simulink model "torqueWalkingMPC"  (Simulink 8.9)
settings: Solver=FixedStepDiscrete  StartTime=0.0  StopTime=Config.t_end  FixedStep=Config.t_step  RelTol=1e-3  EnableMultiTasking=on
InitFcn:
  | cd(fileparts(which(bdroot)));
  | initTorqueWalking;
undefined symbols (not defined in the file or in its folder): biasVectorConstraint_feet, Config, ConstraintMatrix_feet, DiscIntNeverNeededParam, Gains, ROBOT_DOF, Sat
libraries: WBToolboxLibrary x93
(part 3 of 3)

== system torqueWalkingMPC/Dynamics and Kinematics/Inverse Kinematics/QP-Based Inverse Kinematics/inverse kinematics integration ==
  nuDot : Inport
  nu_0 : Inport  Port=2
  q_0 : Inport  Port=3
  Compute Base Pose Derivative : MATLAB Function  TreatAsAtomicUnit=on
  Demux : Demux  Outputs=[7;ROBOT_DOF]
  Demux1 : Demux  Outputs=[6; ROBOT_DOF]
  Demux2 : Demux  Outputs=[16; ROBOT_DOF]
  Integrate nu : DiscreteIntegrator  InitialConditionSource=external  SampleTime=Config.t_step  ICPrevOutput=DiscIntNeverNeededParam  ICPrevScaledInput=DiscIntNeverNeededParam
  Integrate nuDot : DiscreteIntegrator  InitialConditionSource=external  SampleTime=Config.t_step  ICPrevOutput=DiscIntNeverNeededParam  ICPrevScaledInput=DiscIntNeverNeededParam
  Matrix Concatenate : Concatenate  NumInputs=3  Mode=Multidimensional array  ConcatenateDimension=2
  Mux : Mux  Inputs=2
  Mux1 : Mux  Inputs=2
  Mux2 : Mux  Inputs=2
  Reshape : Reshape
  Reshape1 : Reshape  OutputDimensionality=Customize  OutputDimensions=[4;4]
  Rewrite Base Pose as pos+quat : MATLAB Function  TreatAsAtomicUnit=on
  Rewrite Base Pose as transformation matrix : MATLAB Function  TreatAsAtomicUnit=on
  Selector3 : Selector  InputPortWidth=ROBOT_DOF+6  IndexOptions=Index vector (dialog)  Indices=[7:ROBOT_DOF+6]  OutputSizes=1
  Selector4 : Selector  InputPortWidth=ROBOT_DOF+6  IndexOptions=Index vector (dialog)  Indices=[7:ROBOT_DOF+6]  OutputSizes=1
  nu : Outport
  q : Outport  Port=2
  s_sDot_sDDot_des : Outport  Port=3
  wires:
  nu_0/1 -> Integrate nuDot/2
  nuDot/1 -> Selector4/1, Integrate nuDot/1
  Demux/1 -> Rewrite Base Pose as transformation matrix/1(pose_b), Compute Base Pose Derivative/1(pose_b)
  Integrate nu/1 -> Demux/1
  Compute Base Pose Derivative/1(pose_bDot) -> Mux/1
  Demux1/2 -> Mux/2
  Matrix Concatenate/1 -> s_sDot_sDDot_des/1
  Selector3/1 -> Matrix Concatenate/2
  Selector4/1 -> Matrix Concatenate/3
  Demux/2 -> Matrix Concatenate/1, Mux1/2
  Mux/1 -> Integrate nu/1
  Integrate nuDot/1 -> Selector3/1, nu/1, Demux1/1
  Rewrite Base Pose as transformation matrix/1(w_H_b) -> Reshape/1
  Reshape/1 -> Mux1/1
  Mux1/1 -> q/1
  Demux1/1 -> Compute Base Pose Derivative/2(nu_b)
  q_0/1 -> Demux2/1
  Demux2/1 -> Reshape1/1
  Reshape1/1 -> Rewrite Base Pose as pos+quat/1(w_H_b_0)
  Rewrite Base Pose as pos+quat/1(pose_b_0) -> Mux2/1
  Demux2/2 -> Mux2/2
  Mux2/1 -> Integrate nu/2

== system torqueWalkingMPC/Dynamics and Kinematics/Task Accelerations/ComputeTasksPoseAndVelocity/Task position and orientation ==
  s : Inport
  w_H_b : Inport  Port=2
  CoM : WBToolboxLibrary/wholeBodyModel/Kinematics/Forward Kinematics  frameName=Frames.COM  robotName=WBT_robotName  localName=WBT_modelName  wbiFile=WBT_wbiFilename  wbiList=WBT_wbiList
  LFoot : WBToolboxLibrary/wholeBodyModel/Kinematics/Forward Kinematics  frameName=Frames.LEFT_FOOT  robotName=WBT_robotName  localName=WBT_modelName  wbiFile=WBT_wbiFilename  wbiList=WBT_wbiList
  RFoot : WBToolboxLibrary/wholeBodyModel/Kinematics/Forward Kinematics  frameName=Frames.RIGHT_FOOT  robotName=WBT_robotName  localName=WBT_modelName  wbiFile=WBT_wbiFilename  wbiList=WBT_wbiList
  rotational task : WBToolboxLibrary/wholeBodyModel/Kinematics/Forward Kinematics  frameName=Frames.ROT_TASK_LINK  robotName=WBT_robotName  localName=WBT_modelName  wbiFile=WBT_wbiFilename  wbiList=WBT_wbiList
  w_H_CoM : Outport
  w_H_l_sole : Outport  Port=2
  w_H_r_sole : Outport  Port=3
  w_H_rot_task : Outport  Port=4
  wires:
  s/1 -> rotational task/2, RFoot/2, LFoot/2, CoM/2
  w_H_b/1 -> rotational task/1, CoM/1, LFoot/1, RFoot/1
  CoM/1 -> w_H_CoM/1
  LFoot/1 -> w_H_l_sole/1
  RFoot/1 -> w_H_r_sole/1
  rotational task/1 -> w_H_rot_task/1

== system torqueWalkingMPC/Robot State and References/Smooth References /Smooth Reference Orientations/Compose Smoothed References ==
  omegaDot_LFoot : Inport
  omegaDot_RFoot : Inport  Port=2
  omegaDot_rot_task : Inport  Port=3
  w_R_rot_task : Inport  Port=4
  w_R_RFoot : Inport  Port=5
  w_R_LFoot : Inport  Port=6
  omega_LFoot : Inport  Port=7
  omega_RFoot : Inport  Port=8
  omega_rot_task : Inport  Port=9
  Matrix Concatenate1 : Concatenate  NumInputs=3  Mode=Multidimensional array  ConcatenateDimension=2
  Matrix Concatenate2 : Concatenate  NumInputs=3  Mode=Multidimensional array  ConcatenateDimension=2
  Matrix Concatenate6 : Concatenate  NumInputs=3  Mode=Multidimensional array  ConcatenateDimension=2
  orient_vel_acc_LFoot_des : Outport
  orient_vel_acc_RFoot_des : Outport  Port=2
  orient_vel_acc_rot_task_des : Outport  Port=3
  wires:
  w_R_LFoot/1 -> Matrix Concatenate6/1
  Matrix Concatenate6/1 -> orient_vel_acc_LFoot_des/1
  Matrix Concatenate2/1 -> orient_vel_acc_rot_task_des/1
  Matrix Concatenate1/1 -> orient_vel_acc_RFoot_des/1
  omega_LFoot/1 -> Matrix Concatenate6/2
  omegaDot_LFoot/1 -> Matrix Concatenate6/3
  omegaDot_RFoot/1 -> Matrix Concatenate1/3
  omega_RFoot/1 -> Matrix Concatenate1/2
  w_R_RFoot/1 -> Matrix Concatenate1/1
  omegaDot_rot_task/1 -> Matrix Concatenate2/3
  omega_rot_task/1 -> Matrix Concatenate2/2
  w_R_rot_task/1 -> Matrix Concatenate2/1

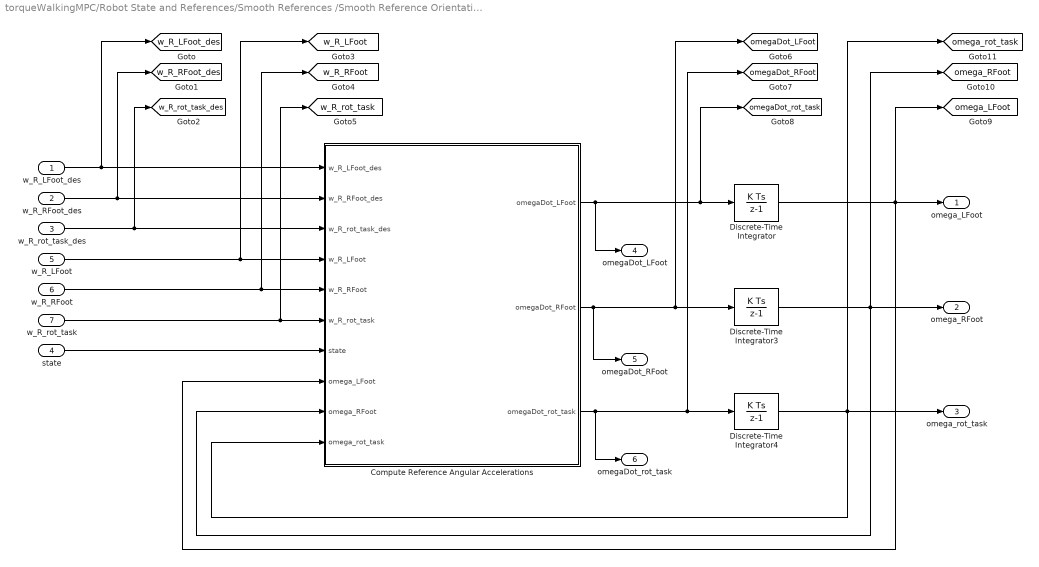
== system torqueWalkingMPC/Robot State and References/Smooth References /Smooth Reference Orientations/Compute Ref Ang Velocities and Accelerations ==
  w_R_LFoot_des : Inport
  w_R_RFoot_des : Inport  Port=2
  w_R_rot_task_des : Inport  Port=3
  state : Inport  Port=4
  w_R_LFoot : Inport  Port=5
  w_R_RFoot : Inport  Port=6
  w_R_rot_task : Inport  Port=7
  Compute Reference Angular Accelerations : MATLAB Function  TreatAsAtomicUnit=on
  Discrete-Time Integrator : DiscreteIntegrator  InitialCondition=zeros(3,1)  InitialConditionSetting=State (most efficient)  SampleTime=Config.t_step  ICPrevOutput=DiscIntNeverNeededParam  ICPrevScaledInput=DiscIntNeverNeededParam
  Discrete-Time Integrator3 : DiscreteIntegrator  InitialCondition=zeros(3,1)  InitialConditionSetting=State (most efficient)  SampleTime=Config.t_step  ICPrevOutput=DiscIntNeverNeededParam  ICPrevScaledInput=DiscIntNeverNeededParam
  Discrete-Time Integrator4 : DiscreteIntegrator  InitialCondition=zeros(3,1)  InitialConditionSetting=State (most efficient)  SampleTime=Config.t_step  ICPrevOutput=DiscIntNeverNeededParam  ICPrevScaledInput=DiscIntNeverNeededParam
  omega_LFoot : Outport
  omega_RFoot : Outport  Port=2
  omega_rot_task : Outport  Port=3
  omegaDot_LFoot : Outport  Port=4
  omegaDot_RFoot : Outport  Port=5
  omegaDot_rot_task : Outport  Port=6
  tag scope: omegaDot_LFoot=global, omegaDot_RFoot=global, omegaDot_rot_task=global, omega_LFoot=global, omega_RFoot=global, omega_rot_task=global, w_R_LFoot=global, w_R_LFoot_des=global, w_R_RFoot=global, w_R_RFoot_des=global, w_R_rot_task=global, w_R_rot_task_des=global
  wires:
  w_R_RFoot/1 -> [w_R_RFoot], Compute Reference Angular Accelerations/5(w_R_RFoot)
  w_R_rot_task/1 -> [w_R_rot_task], Compute Reference Angular Accelerations/6(w_R_rot_task)
  w_R_LFoot/1 -> [w_R_LFoot], Compute Reference Angular Accelerations/4(w_R_LFoot)
  Compute Reference Angular Accelerations/1(omegaDot_LFoot) -> [omegaDot_rot_task], Discrete-Time Integrator/1, omegaDot_LFoot/1
  Compute Reference Angular Accelerations/3(omegaDot_rot_task) -> [omegaDot_RFoot], Discrete-Time Integrator4/1, omegaDot_rot_task/1
  Compute Reference Angular Accelerations/2(omegaDot_RFoot) -> [omegaDot_LFoot], Discrete-Time Integrator3/1, omegaDot_RFoot/1
  w_R_LFoot_des/1 -> [w_R_LFoot_des], Compute Reference Angular Accelerations/1(w_R_LFoot_des)
  w_R_RFoot_des/1 -> [w_R_RFoot_des], Compute Reference Angular Accelerations/2(w_R_RFoot_des)
  w_R_rot_task_des/1 -> [w_R_rot_task_des], Compute Reference Angular Accelerations/3(w_R_rot_task_des)
  state/1 -> Compute Reference Angular Accelerations/7(state)
  Discrete-Time Integrator4/1 -> Compute Reference Angular Accelerations/10(omega_rot_task), omega_rot_task/1, [omega_rot_task]
  Discrete-Time Integrator3/1 -> omega_RFoot/1, [omega_RFoot], Compute Reference Angular Accelerations/9(omega_RFoot)
  Discrete-Time Integrator/1 -> [omega_LFoot], Compute Reference Angular Accelerations/8(omega_LFoot), omega_LFoot/1

== system torqueWalkingMPC/Robot State and References/Smooth References /Smooth Reference Orientations/Compute Smoothed Ref Orientations ==
  w_R_LFoot_des : Inport
  w_R_RFoot_des : Inport  Port=2
  w_R_rot_task_des : Inport  Port=3
  omega_LFoot : Inport  Port=4
  omega_RFoot : Inport  Port=5
  omega_rot_task : Inport  Port=6
  Compute Rotation Matrix Derivative : MATLAB Function  TreatAsAtomicUnit=on
  Discrete-Time Integrator1 : DiscreteIntegrator  InitialConditionSource=external  InitialCondition=zeros(3,1)  InitialConditionSetting=State (most efficient)  SampleTime=Config.t_step  ICPrevOutput=DiscIntNeverNeededParam  ICPrevScaledInput=DiscIntNeverNeededParam
  Discrete-Time Integrator2 : DiscreteIntegrator  InitialConditionSource=external  InitialCondition=zeros(3,1)  InitialConditionSetting=State (most efficient)  SampleTime=Config.t_step  ICPrevOutput=DiscIntNeverNeededParam  ICPrevScaledInput=DiscIntNeverNeededParam
  Discrete-Time Integrator5 : DiscreteIntegrator  InitialConditionSource=external  InitialCondition=zeros(3,1)  InitialConditionSetting=State (most efficient)  SampleTime=Config.t_step  ICPrevOutput=DiscIntNeverNeededParam  ICPrevScaledInput=DiscIntNeverNeededParam
  "holder " : WBToolboxLibrary/Utilities/holder 
  holder 1 : WBToolboxLibrary/Utilities/holder 
  holder 2 : WBToolboxLibrary/Utilities/holder 
  w_R_LFoot : Outport
  w_R_RFoot : Outport  Port=2
  w_R_rot_task : Outport  Port=3
  wires:
  "holder "/1 -> Discrete-Time Integrator2/2
  holder 2/1 -> Discrete-Time Integrator5/2
  holder 1/1 -> Discrete-Time Integrator1/2
  Compute Rotation Matrix Derivative/1(RDot_LFoot) -> Discrete-Time Integrator2/1
  Compute Rotation Matrix Derivative/2(RDot_RFoot) -> Discrete-Time Integrator5/1
  Compute Rotation Matrix Derivative/3(RDot_rot_task) -> Discrete-Time Integrator1/1
  w_R_LFoot_des/1 -> "holder "/1
  w_R_RFoot_des/1 -> holder 2/1
  w_R_rot_task_des/1 -> holder 1/1
  Discrete-Time Integrator2/1 -> w_R_LFoot/1, Compute Rotation Matrix Derivative/4(w_R_LFoot)
  Discrete-Time Integrator1/1 -> w_R_rot_task/1, Compute Rotation Matrix Derivative/6(w_R_rot_task)
  omega_LFoot/1 -> Compute Rotation Matrix Derivative/1(omega_LFoot)
  omega_RFoot/1 -> Compute Rotation Matrix Derivative/2(omega_RFoot)
  omega_rot_task/1 -> Compute Rotation Matrix Derivative/3(omega_rot_task)
  Discrete-Time Integrator5/1 -> w_R_RFoot/1, Compute Rotation Matrix Derivative/5(w_R_RFoot)

== system torqueWalkingMPC/Robot State and References/State Machines/Compute Feet to Base Link Transforms/LFoot to base link transform  ==
  s : Inport
  inertial : Inport  Port=2
  w_H_link : Inport  Port=3
  w_H_base_fixed : Inport  Port=4
  Fixed base to imu transform : WBToolboxLibrary/wholeBodyModel/Kinematics/Forward Kinematics  frameName=Frames.IMU  robotName=WBT_robotName  localName=WBT_modelName  wbiFile=WBT_wbiFilename  wbiList=WBT_wbiList
  Fixed base to root link transform : WBToolboxLibrary/wholeBodyModel/Kinematics/Forward Kinematics  frameName=Frames.BASE_LINK  robotName=WBT_robotName  localName=WBT_modelName  wbiFile=WBT_wbiFilename  wbiList=WBT_wbiList
  Inv\* : Product  Inputs=/*  Multiplication=Matrix(*)
  "Inv\\*  " : Product  Inputs=/*  Multiplication=Matrix(*)
  Neck Position : WBToolboxLibrary/Utilities/Yarp Read  portName=Ports.NECK_POS  signalSize=6  blocking=off  timestamp=off  autoconnect=on  errorOnConnection=off
  Switch6 : Switch  Criteria=u2 > Threshold
  USE_IMU4EST_BASE : Constant  Value=Config.USE_IMU4EST_BASE
  fromImuToHomogeousTransformFCN : MATLAB Function  TreatAsAtomicUnit=on
  holder 1 : WBToolboxLibrary/Utilities/holder 
  holder 2 : WBToolboxLibrary/Utilities/holder 
  neck transform : Subsystem
  link_H_b : Outport
  wires:
  Switch6/1 -> link_H_b/1
  "Inv\\*  "/1 -> Switch6/3, fromImuToHomogeousTransformFCN/3(link_H_base)  "link_H_root"
  USE_IMU4EST_BASE/1 -> Switch6/2
  Inv\*/1 -> fromImuToHomogeousTransformFCN/1(imu_H_link), holder 1/1  "imu_H_link"
  holder 2/1 -> fromImuToHomogeousTransformFCN/4(inertial_0)
  Fixed base to imu transform/1 -> Inv\*/1
  holder 1/1 -> fromImuToHomogeousTransformFCN/2(imu_H_link_0)
  s/1 -> Fixed base to imu transform/2, Fixed base to root link transform/2
  fromImuToHomogeousTransformFCN/1(w_H_b) -> Switch6/1
  Fixed base to root link transform/1 -> "Inv\\*  "/2
  inertial/1 -> holder 2/1, fromImuToHomogeousTransformFCN/5(inertial)
  Neck Position/1 -> neck transform/1(neck port)
  neck transform/1(neck position) -> fromImuToHomogeousTransformFCN/6(neck_pos)
  w_H_link/1 -> "Inv\\*  "/1, Inv\*/2
  w_H_base_fixed/1 -> Fixed base to root link transform/1, Fixed base to imu transform/1

== system torqueWalkingMPC/Robot State and References/State Machines/Compute Feet to Base Link Transforms/RFoot to base link transform ==
  s : Inport
  inertial : Inport  Port=2
  w_H_link : Inport  Port=3
  w_H_base_fixed : Inport  Port=4
  Fixed base to imu transform : WBToolboxLibrary/wholeBodyModel/Kinematics/Forward Kinematics  frameName=Frames.IMU  robotName=WBT_robotName  localName=WBT_modelName  wbiFile=WBT_wbiFilename  wbiList=WBT_wbiList
  Fixed base to root link transform : WBToolboxLibrary/wholeBodyModel/Kinematics/Forward Kinematics  frameName=Frames.BASE_LINK  robotName=WBT_robotName  localName=WBT_modelName  wbiFile=WBT_wbiFilename  wbiList=WBT_wbiList
  Inv\* : Product  Inputs=/*  Multiplication=Matrix(*)
  "Inv\\*  " : Product  Inputs=/*  Multiplication=Matrix(*)
  Neck Position : WBToolboxLibrary/Utilities/Yarp Read  portName=Ports.NECK_POS  signalSize=6  blocking=off  timestamp=off  autoconnect=on  errorOnConnection=off
  Switch6 : Switch  Criteria=u2 > Threshold
  USE_IMU4EST_BASE : Constant  Value=Config.USE_IMU4EST_BASE
  fromImuToHomogeousTransformFCN : MATLAB Function  TreatAsAtomicUnit=on
  holder 1 : WBToolboxLibrary/Utilities/holder 
  holder 2 : WBToolboxLibrary/Utilities/holder 
  neck transform : Subsystem
  link_H_b : Outport
  wires:
  Switch6/1 -> link_H_b/1
  "Inv\\*  "/1 -> Switch6/3, fromImuToHomogeousTransformFCN/3(link_H_base)  "link_H_root"
  USE_IMU4EST_BASE/1 -> Switch6/2
  Inv\*/1 -> fromImuToHomogeousTransformFCN/1(imu_H_link), holder 1/1  "imu_H_link"
  holder 2/1 -> fromImuToHomogeousTransformFCN/4(inertial_0)
  Fixed base to imu transform/1 -> Inv\*/1
  holder 1/1 -> fromImuToHomogeousTransformFCN/2(imu_H_link_0)
  s/1 -> Fixed base to imu transform/2, Fixed base to root link transform/2
  fromImuToHomogeousTransformFCN/1(w_H_b) -> Switch6/1
  Fixed base to root link transform/1 -> "Inv\\*  "/2
  inertial/1 -> holder 2/1, fromImuToHomogeousTransformFCN/5(inertial)
  Neck Position/1 -> neck transform/1(neck port)
  neck transform/1(neck position) -> fromImuToHomogeousTransformFCN/6(neck_pos)
  w_H_link/1 -> "Inv\\*  "/1, Inv\*/2
  w_H_base_fixed/1 -> Fixed base to root link transform/1, Fixed base to imu transform/1

== system torqueWalkingMPC/Robot State and References/State Machines/Compute State Velocity/Feet Jacobians ==
  s : Inport
  w_H_b : Inport  Port=2
  Jacobian LFoot : WBToolboxLibrary/wholeBodyModel/Jacobians/Jacobian  frameName=Frames.LEFT_FOOT  robotName=WBT_robotName  localName=WBT_modelName  wbiFile=WBT_wbiFilename  wbiList=WBT_wbiList
  Jacobian RFoot : WBToolboxLibrary/wholeBodyModel/Jacobians/Jacobian  frameName=Frames.RIGHT_FOOT  robotName=WBT_robotName  localName=WBT_modelName  wbiFile=WBT_wbiFilename  wbiList=WBT_wbiList
  J_LFoot : Outport
  J_RFoot : Outport  Port=2
  wires:
  Jacobian LFoot/1 -> J_LFoot/1
  Jacobian RFoot/1 -> J_RFoot/1
  w_H_b/1 -> Jacobian RFoot/1, Jacobian LFoot/1
  s/1 -> Jacobian LFoot/2, Jacobian RFoot/2

== system torqueWalkingMPC/Robot State and References/State Machines/Select the Current State and References/task position and orientation ==
  s : Inport
  w_H_b : Inport  Port=2
  CoM : WBToolboxLibrary/wholeBodyModel/Kinematics/Forward Kinematics  frameName=Frames.COM  robotName=WBT_robotName  localName=WBT_modelName  wbiFile=WBT_wbiFilename  wbiList=WBT_wbiList
  LFoot : WBToolboxLibrary/wholeBodyModel/Kinematics/Forward Kinematics  frameName=Frames.LEFT_FOOT  robotName=WBT_robotName  localName=WBT_modelName  wbiFile=WBT_wbiFilename  wbiList=WBT_wbiList
  RFoot : WBToolboxLibrary/wholeBodyModel/Kinematics/Forward Kinematics  frameName=Frames.RIGHT_FOOT  robotName=WBT_robotName  localName=WBT_modelName  wbiFile=WBT_wbiFilename  wbiList=WBT_wbiList
  rotational task : WBToolboxLibrary/wholeBodyModel/Kinematics/Forward Kinematics  frameName=Frames.ROT_TASK_LINK  robotName=WBT_robotName  localName=WBT_modelName  wbiFile=WBT_wbiFilename  wbiList=WBT_wbiList
  w_H_CoM : Outport
  w_H_l_sole : Outport  Port=2
  w_H_r_sole : Outport  Port=3
  w_H_rot_task : Outport  Port=4
  wires:
  s/1 -> rotational task/2, RFoot/2, LFoot/2, CoM/2
  w_H_b/1 -> rotational task/1, CoM/1, LFoot/1, RFoot/1
  CoM/1 -> w_H_CoM/1
  LFoot/1 -> w_H_l_sole/1
  RFoot/1 -> w_H_r_sole/1
  rotational task/1 -> w_H_rot_task/1

== system torqueWalkingMPC/Robot State and References/State Machines/Compute Feet to Base Link Transforms/LFoot to base link transform /neck transform ==
  neck port : Inport
  Constant : Constant  Value=zeros(3,1)
  Gain : Gain  Gain=pi/180
  Selector1 : Selector  InputPortWidth=6  IndexOptions=Index vector (dialog)  Indices=[1:3]  OutputSizes=1
  Switch : Switch  Criteria=u2 > Threshold
  USE_IMU4EST_BASE1 : Constant  Value=Config.CORRECT_IMU_WITH_NECK_POS
  neck position : Outport
  wires:
  neck port/1 -> Gain/1
  USE_IMU4EST_BASE1/1 -> Switch/2
  Switch/1 -> neck position/1
  Gain/1 -> Selector1/1
  Constant/1 -> Switch/3
  Selector1/1 -> Switch/1  "neck pos"

== system torqueWalkingMPC/Robot State and References/State Machines/Compute Feet to Base Link Transforms/RFoot to base link transform/neck transform ==
  neck port : Inport
  Constant : Constant  Value=zeros(3,1)
  Gain : Gain  Gain=pi/180
  Selector1 : Selector  InputPortWidth=6  IndexOptions=Index vector (dialog)  Indices=[1:3]  OutputSizes=1
  Switch : Switch  Criteria=u2 > Threshold
  USE_IMU4EST_BASE1 : Constant  Value=Config.CORRECT_IMU_WITH_NECK_POS
  neck position : Outport
  wires:
  neck port/1 -> Gain/1
  USE_IMU4EST_BASE1/1 -> Switch/2
  Switch/1 -> neck position/1
  Gain/1 -> Selector1/1
  Constant/1 -> Switch/3
  Selector1/1 -> Switch/1  "neck pos"

== matlab function Dynamics and Kinematics/Initial Conditions/compute state velocity/Compute Base Velocity ==
  data: J_LeftFoot input double; J_RightFoot input double; feetInContact input double; nu_b output double; sDot input double; Sat parameter double
function nu_b = computeBaseVelocityFCN(J_LeftFoot, J_RightFoot, feetInContact, sDot, Sat)

    nu_b = computeBaseVelocity(J_LeftFoot, J_RightFoot, feetInContact, sDot, Sat);
end

== matlab function Balancing Controller (Reactive QP control)/Balancing Controller Function ==
  data: feetInContact input double; M input double; Hessian output double; h input double; J input double; impedances input double; dampings input double; s input double; sDot input double; s_sDot_sDDot_des input double; acc_task_star input double; JDot_nu input double; ConstraintsMatrix_feet input double; biasVectorConstraint_feet input double; w_H_l_sole input double; w_H_r_sole input double; gradient output double; ConstraintMatrix_equality output double; biasVectorConstraint_equality output double; ConstraintMatrix_inequality output double; biasVectorConstraint_inequality output double; Sat parameter double; Config parameter double
function [Hessian,gradient,ConstraintMatrix_equality,biasVectorConstraint_equality, ...
          ConstraintMatrix_inequality,biasVectorConstraint_inequality] = ...
          balancingControllerFCN(feetInContact, M, h, J, impedances, ...
                                 dampings, s, sDot, s_sDot_sDDot_des, acc_task_star, ...
                                 JDot_nu, ConstraintsMatrix_feet, biasVectorConstraint_feet, ...
                                 w_H_l_sole, w_H_r_sole, Sat, Config)
                          

    [Hessian,gradient,ConstraintMatrix_equality,biasVectorConstraint_equality, ...
     ConstraintMatrix_inequality,biasVectorConstraint_inequality] = ...
         balancingControllerMPC(feetInContact, M, h, J, impedances, ...
                                dampings, s, sDot, s_sDot_sDDot_des, acc_task_star, ...
                                JDot_nu, ConstraintsMatrix_feet, biasVectorConstraint_feet, ...
                                w_H_l_sole, w_H_r_sole, Sat, Config);                         
end

== matlab function Dynamics and Kinematics/Inverse Kinematics/Compute tasks accelerations ==
  data: pos_vel_acc_CoM_des input double; acc_task_star output double; pose_vel_acc_LFoot_des input double; pose_vel_acc_RFoot_des input double; orient_vel_acc_rot_task_des input double; pos_vel_CoM input double; pose_vel_LFoot input double; pose_vel_RFoot input double; orient_vel_rot_task input double; Kp_Kd_CoM input double; Kp_Kd_LFoot input double; Kp_Kd_RFoot input double; Kp_Kd_rot_task input double; feetInContact input double; Sat parameter double
function acc_task_star = setTasksAccelerationsFCN(pos_vel_acc_CoM_des,pose_vel_acc_LFoot_des,pose_vel_acc_RFoot_des,orient_vel_acc_rot_task_des, ...
                                                  pos_vel_CoM, pose_vel_LFoot, pose_vel_RFoot, orient_vel_rot_task, ...
                                                  Kp_Kd_CoM, Kp_Kd_LFoot, Kp_Kd_RFoot, Kp_Kd_rot_task, feetInContact, Sat) 

    acc_task_star = setTasksAccelerations(pos_vel_acc_CoM_des,pose_vel_acc_LFoot_des,pose_vel_acc_RFoot_des,orient_vel_acc_rot_task_des, ...
                                          pos_vel_CoM, pose_vel_LFoot, pose_vel_RFoot, orient_vel_rot_task, ...
                                          Kp_Kd_CoM, Kp_Kd_LFoot, Kp_Kd_RFoot, Kp_Kd_rot_task, feetInContact, Sat);   
end

== matlab function Dynamics and Kinematics/Inverse Kinematics/ComputeTasksPoseAndVelocity/Compose Task Pose and Velocity ==
  data: vel_CoM input double; vel_LFoot input double; vel_RFoot input double; vel_rot_task input double; pos_vel_CoM output double; pose_vel_LFoot output double; pose_vel_RFoot output double; orient_vel_rot_task output double; w_H_CoM input double; w_H_l_sole input double; w_H_r_sole input double; w_H_rot_task input double
function [pos_vel_CoM, pose_vel_LFoot, pose_vel_RFoot, orient_vel_rot_task] = ...
             composeTaskPoseAndVelocityFCN(vel_CoM, vel_LFoot, vel_RFoot, vel_rot_task, ...
                                           w_H_CoM, w_H_l_sole, w_H_r_sole, w_H_rot_task)
                                                                                                                              
    [pos_vel_CoM, pose_vel_LFoot, pose_vel_RFoot, orient_vel_rot_task] = ...
       composeTaskPoseAndVelocity(vel_CoM, vel_LFoot, vel_RFoot, vel_rot_task, ...
                                  w_H_CoM, w_H_l_sole, w_H_r_sole, w_H_rot_task);
end

== matlab function Dynamics and Kinematics/Inverse Kinematics/QP-Based Inverse Kinematics/Compute QP Hessian, gradient and constraints  ==
  data: s input double; nu input double; s_sDot_sDDot_ref input double; Hessian output double; impedances input double; dampings input double; J input double; JDot_nu input double; acc_task_star input double; gradient output double; ConstraintMatrix output double; biasVectorConstraint output double
function [Hessian, gradient, ConstraintMatrix, biasVectorConstraint] = ...
             computeQPHessianAndConstraintsFCN(s, nu, s_sDot_sDDot_ref, impedances, dampings, J, JDot_nu, acc_task_star)
    
    [Hessian, gradient, ConstraintMatrix, biasVectorConstraint] = ...
        computeQPHessianAndConstraints(s, nu, s_sDot_sDDot_ref, impedances, dampings, J, JDot_nu, acc_task_star);
end

== matlab function Dynamics and Kinematics/Task Accelerations/Compute tasks accelerations ==
  data: pos_vel_acc_CoM_des input double; acc_task_star output double; pose_vel_acc_LFoot_des input double; pose_vel_acc_RFoot_des input double; orient_vel_acc_rot_task_des input double; pos_vel_CoM input double; pose_vel_LFoot input double; pose_vel_RFoot input double; orient_vel_rot_task input double; Kp_Kd_CoM input double; Kp_Kd_LFoot input double; Kp_Kd_RFoot input double; Kp_Kd_rot_task input double; feetInContact input double; Sat parameter double
function acc_task_star = setTasksAccelerationsFCN(pos_vel_acc_CoM_des,pose_vel_acc_LFoot_des,pose_vel_acc_RFoot_des,orient_vel_acc_rot_task_des, ...
                                                  pos_vel_CoM, pose_vel_LFoot, pose_vel_RFoot, orient_vel_rot_task, ...
                                                  Kp_Kd_CoM, Kp_Kd_LFoot, Kp_Kd_RFoot, Kp_Kd_rot_task, feetInContact, Sat) 

    acc_task_star = setTasksAccelerations(pos_vel_acc_CoM_des,pose_vel_acc_LFoot_des,pose_vel_acc_RFoot_des,orient_vel_acc_rot_task_des, ...
                                          pos_vel_CoM, pose_vel_LFoot, pose_vel_RFoot, orient_vel_rot_task, ...
                                          Kp_Kd_CoM, Kp_Kd_LFoot, Kp_Kd_RFoot, Kp_Kd_rot_task, feetInContact, Sat); 
end

== matlab function Dynamics and Kinematics/Task Accelerations/ComputeTasksPoseAndVelocity/Compose Task Pose and Velocity ==
  data: vel_CoM input double; vel_LFoot input double; vel_RFoot input double; vel_rot_task input double; pos_vel_CoM output double; pose_vel_LFoot output double; pose_vel_RFoot output double; orient_vel_rot_task output double; w_H_CoM input double; w_H_l_sole input double; w_H_r_sole input double; w_H_rot_task input double
function [pos_vel_CoM, pose_vel_LFoot, pose_vel_RFoot, orient_vel_rot_task] = ...
             composeTaskPoseAndVelocityFCN(vel_CoM, vel_LFoot, vel_RFoot, vel_rot_task, ...
                                           w_H_CoM, w_H_l_sole, w_H_r_sole, w_H_rot_task)
                                                                                                                              
    [pos_vel_CoM, pose_vel_LFoot, pose_vel_RFoot, orient_vel_rot_task] = ...
        composeTaskPoseAndVelocity(vel_CoM, vel_LFoot, vel_RFoot, vel_rot_task, ...
                                   w_H_CoM, w_H_l_sole, w_H_r_sole, w_H_rot_task);
end

== matlab function Robot State and References/Gain Scheduling/Gain Scheduling Function ==
  data: state input double; Kp_CoM output double; Kd_CoM output double; Kp_LFoot output double; Kd_LFoot output double; Kp_RFoot output double; Kd_RFoot output double; Kp_rot_task output double; Kd_rot_task output double; impedances output double; dampings output double; Gains parameter double; smoothingTimeGains output double; Config parameter double
function [Kp_CoM, Kd_CoM, Kp_LFoot, Kd_LFoot, Kp_RFoot, Kd_RFoot, Kp_rot_task, Kd_rot_task, impedances, dampings, smoothingTimeGains] = ...
             gainSchedulingFCN(state,Gains,Config)

    [Kp_CoM, Kd_CoM, Kp_LFoot, Kd_LFoot, Kp_RFoot, Kd_RFoot, Kp_rot_task, Kd_rot_task, impedances, dampings, smoothingTimeGains] = ...
        gainScheduling(state,Gains,Config);
end

== matlab function Robot State and References/Smooth References /Smooth Reference Orientations/Compute Ref Ang Velocities and Accelerations/Compute Reference Angular Accelerations ==
  data: w_R_LFoot_des input double; w_R_RFoot_des input double; w_R_rot_task_des input double; w_R_LFoot input double; w_R_RFoot input double; omegaDot_LFoot output double; omegaDot_RFoot output double; omegaDot_rot_task output double; w_R_rot_task input double; state input double; omega_LFoot input double; omega_RFoot input double; omega_rot_task input double; Config parameter double
function [omegaDot_LFoot, omegaDot_RFoot, omegaDot_rot_task] = computeRefAngAccelerationFCN(w_R_LFoot_des, w_R_RFoot_des, w_R_rot_task_des, ...
                                                                                            w_R_LFoot, w_R_RFoot, w_R_rot_task, ...
                                                                                            state, omega_LFoot, omega_RFoot, omega_rot_task, Config)
         
    % Compute reference angular accelerations given a desired rotation matrix
    omegaDot_LFoot     = rotationalPID(w_R_LFoot, omega_LFoot, w_R_LFoot_des, zeros(3,1), zeros(3,1), ...
                                       Config.LFoot_Kp_smoothing(state), Config.LFoot_Kd_smoothing(state));
                                   
    omegaDot_RFoot     = rotationalPID(w_R_RFoot, omega_RFoot, w_R_RFoot_des, zeros(3,1), zeros(3,1), ...
                                       Config.RFoot_Kp_smoothing(state), Config.RFoot_Kd_smoothing(state));
                                   
    omegaDot_rot_task  = rotationalPID(w_R_rot_task, omega_rot_task, w_R_rot_task_des, zeros(3,1), zeros(3,1), ...
                                       Config.rot_task_Kp_smoothing(state), Config.rot_task_Kd_smoothing(state));
end

== matlab function Robot State and References/State Machines/Select the Current State and References/STATE MACHINES ==
  data: s_0 input double; w_H_CoM_0 input double; w_H_LFoot_0 input double; w_H_RFoot_0 input double; w_H_rot_task_0 input double; LFoot_H_b input double; RFoot_H_b input double; t input double; LFoot_wrench input double; RFoot_wrench input double; state output double; references_CoM output double; references_LFoot output double; references_RFoot output double; references_rot_task output double; feetInContact output double; references_s output double; w_H_b output double; Config parameter double
function [state, references_CoM, references_LFoot, references_RFoot, references_rot_task, feetInContact, references_s, w_H_b] = stateMachinesFCN ...
             (s_0, w_H_CoM_0, w_H_LFoot_0, w_H_RFoot_0, w_H_rot_task_0, LFoot_H_b, RFoot_H_b, ... 
              t, LFoot_wrench, RFoot_wrench, Config)

    [state, references_CoM, references_LFoot, references_RFoot, references_rot_task, feetInContact, references_s, w_H_b] = stateMachineExample ...
        (s_0, w_H_CoM_0, w_H_LFoot_0, w_H_RFoot_0, w_H_rot_task_0, t, LFoot_H_b, RFoot_H_b, LFoot_wrench, RFoot_wrench, Config);

end

== matlab function Robot State and References/State Machines/Compute Feet to Base Link Transforms/LFoot to base link transform /fromImuToHomogeousTransformFCN ==
  data: imu_H_link input double; imu_H_link_0 input double; link_H_base input double; inertial_0 input double; inertial input double; neck_pos input double; w_H_b output double; Config parameter double
function w_H_b = worldToBaseTransformWithIMUFCN(imu_H_link,imu_H_link_0,link_H_base,inertial_0,inertial,neck_pos,Config)

    w_H_b = worldToBaseTransformWithIMU(imu_H_link,imu_H_link_0,link_H_base,inertial_0,inertial,neck_pos,Config);

end

== matlab function Robot State and References/Smooth References /Smooth Reference Orientations/Compute Smoothed Ref Orientations/Compute Rotation Matrix Derivative ==
  data: RDot_LFoot output double; RDot_RFoot output double; RDot_rot_task output double; omega_LFoot input double; omega_RFoot input double; omega_rot_task input double; w_R_LFoot input double; w_R_RFoot input double; w_R_rot_task input double
function [RDot_LFoot, RDot_RFoot, RDot_rot_task] = rotationDerivativeFromAngVelFCN(omega_LFoot, omega_RFoot, omega_rot_task, ... 
                                                                                   w_R_LFoot, w_R_RFoot, w_R_rot_task)
         
    % Compute the rotation matrix derivative given the angular velocity
    RDot_LFoot     = rotationDerivativeFromAngVel(omega_LFoot,w_R_LFoot);
    RDot_RFoot     = rotationDerivativeFromAngVel(omega_RFoot,w_R_RFoot);
    RDot_rot_task  = rotationDerivativeFromAngVel(omega_rot_task, w_R_rot_task);      
end

== matlab function Robot State and References/State Machines/Compute Feet to Base Link Transforms/RFoot to base link transform/fromImuToHomogeousTransformFCN ==
  data: imu_H_link input double; imu_H_link_0 input double; link_H_base input double; inertial_0 input double; inertial input double; neck_pos input double; w_H_b output double; Config parameter double
function w_H_b = worldToBaseTransformWithIMUFCN(imu_H_link,imu_H_link_0,link_H_base,inertial_0,inertial,neck_pos,Config)

    w_H_b = worldToBaseTransformWithIMU(imu_H_link,imu_H_link_0,link_H_base,inertial_0,inertial,neck_pos,Config);

end

== matlab function Robot State and References/State Machines/Compute State Velocity/Compute Base Velocity ==
  data: J_LeftFoot input double; J_RightFoot input double; feetInContact input double; nu_b output double; sDot input double; Sat parameter double
function nu_b = computeBaseVelocityFCN(J_LeftFoot, J_RightFoot, feetInContact, sDot, Sat)

    nu_b = computeBaseVelocity(J_LeftFoot, J_RightFoot, feetInContact, sDot, Sat);
end

== matlab function Dynamics and Kinematics/Inverse Kinematics/QP-Based Inverse Kinematics/inverse kinematics integration/Rewrite Base Pose as transformation matrix ==
  data: pose_b input double; w_H_b output double
function  w_H_b = fromPosQuatToTransfMatrFCN(pose_b) 

    % converts the base pose from a position + quaternion representation 
    % to a tranformation matrix
    w_H_b = fromPosQuatToTransfMatr(pose_b);
end

== matlab function Dynamics and Kinematics/Inverse Kinematics/QP-Based Inverse Kinematics/inverse kinematics integration/Compute Base Pose Derivative ==
  data: pose_b input double; nu_b input double; pose_bDot output double
function pose_bDot = basePoseDerivativeFCN(pose_b,nu_b)

    % time derivative of the floating base pose
    pose_bDot = basePoseDerivative(nu_b, pose_b);
end

== matlab function Robot State and References/Smooth References /Smooth Reference Positions/Configure Settling Times ==
  data: state input double; Config parameter double; smoothingTime_CoM output double; smoothingTime_LFoot output double; smoothingTime_RFoot output double; smoothingTime_joints output double
function [smoothingTime_CoM, smoothingTime_LFoot, smoothingTime_RFoot, smoothingTime_joints] = setSmoothingTimesFCN(state,Config)

    [smoothingTime_CoM, smoothingTime_LFoot, smoothingTime_RFoot, smoothingTime_joints] = setSmoothingTimes(state,Config);

end

== matlab function Dynamics and Kinematics/Inverse Kinematics/QP-Based Inverse Kinematics/inverse kinematics integration/Rewrite Base Pose as pos+quat ==
  data: w_H_b_0 input double; pose_b_0 output double
function pose_b_0 = fromTransfMatrixToPosQuatFCN(w_H_b_0)

    % converts the floating base pose expressed in terms of transformation
    % matrix into position + quaternion representation 
    pose_b_0 = fromTransfMatrixToPosQuat(w_H_b_0);

end

== matlab function Dynamics and Kinematics/Compute Dynamic and Kinematic Quantities/Mass Matrix and Bias Forces/Add motors reflected inertias/Add motor reflected inertias ==
  data: M input double; M_with_inertia output double; Config parameter double
function M_with_inertia = addMotorsInertiaFCN(M,Config)

    M_with_inertia = addMotorsInertia(M,Config);

end
